simulink model "AeroPlantMIAC_2018a"  (Simulink 9.1)
settings: Solver=VariableStepAuto  StartTime=0.0  StopTime=5  FixedStep=0.01  MaxStep=0.01  RelTol=1e-3  EnableMultiTasking=on
values from neighbouring files (symbols this model uses):
  sigma2e = 0.0    (= 0)    [SA_ACex4_SKRYPT.m]
  Ta = 0.005    [SA_ACex4_SKRYPT.m]
  Tc = 0.001    [SA_ACex4_SKRYPT.m]
  Yr = 0.15    [SA_ACex4_SKRYPT.m]
undefined symbols (not defined in the file or in its folder): T, wr
libraries: simulink x1
settings Model: Creator=Gebruiker  LastModifiedBy=Adam
settings DataIOCC: LimitDataPoints=on  SignalLoggingSaveFormat=ModelDataLogs
settings OptimizationCC: InitFltsAndDblsToZero=on
settings DebuggingCC: SaveWithParameterizedLinksMsg=none  SignalResolutionControl=TryResolveAllWithWarning  SolverPrmCheckMsg=warning  MultiTaskDSMMsg=warning  MultiTaskCondExecSysMsg=none  FcnCallInpInsideContextMsg=warning
settings SFSimCC: SimUseLocalCustomCode=on
settings RTWCC: RTWUseLocalCustomCode=on
settings GRTTargetCC: TargetFcnLib=ansi_tfl_tmw.mat
settings ConfigComp: CovExternalEMLEnable=on

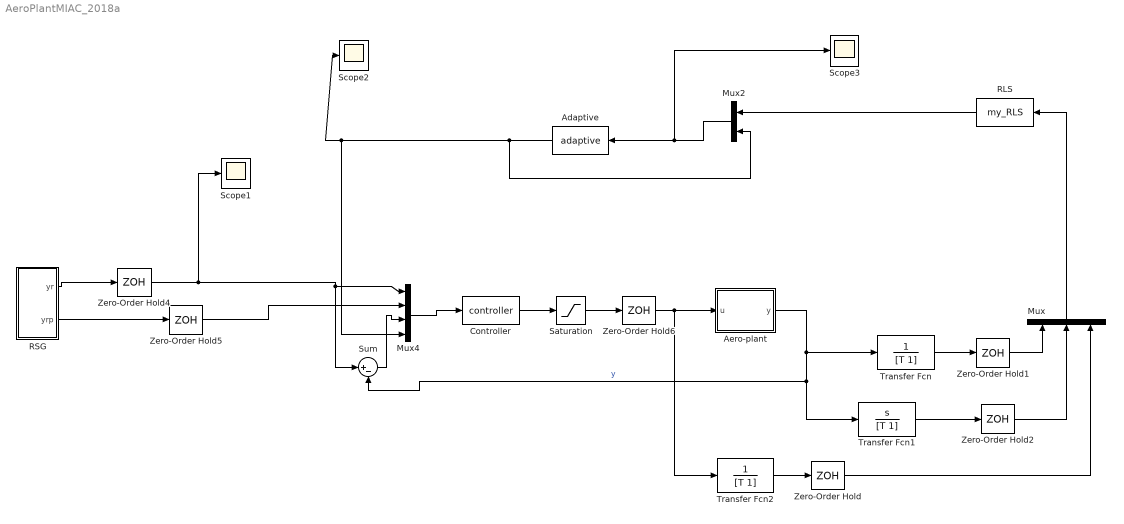
== system AeroPlantMIAC_2018a ==
  Adaptive : MATLABFcn  MATLABFcn=adaptive
  Aero-plant : Subsystem
  Controller : MATLABFcn  MATLABFcn=controller  OutputDimensions=1
  Mux : Mux  Inputs=3
  Mux2 : Mux  Inputs=[2 3]
  Mux4 : Mux
  RLS : MATLABFcn  MATLABFcn=my_RLS  OutputDimensions=2
  RSG : Subsystem
  Saturation : Saturate  UpperLimit=pi/2  LowerLimit=-pi/2
  Scope1 : Scope
  Scope2 : Scope
  Scope3 : Scope
  Sum : Sum  Inputs=|+-
  Transfer Fcn : TransferFcn  Numerator=[0 1]  Denominator=[T 1]
  Transfer Fcn1 : TransferFcn  Numerator=[1 0]  Denominator=[T 1]
  Transfer Fcn2 : TransferFcn  Numerator=[0 1]  Denominator=[T 1]
  Zero-Order Hold : ZeroOrderHold  SampleTime=Ta
  Zero-Order Hold1 : ZeroOrderHold  SampleTime=Ta
  Zero-Order Hold2 : ZeroOrderHold  SampleTime=Ta
  Zero-Order Hold4 : ZeroOrderHold  SampleTime=Tc
  Zero-Order Hold5 : ZeroOrderHold  SampleTime=Tc
  Zero-Order Hold6 : ZeroOrderHold  SampleTime=Tc
  wires:
  Aero-plant/1(y) -> Transfer Fcn1/1, Sum/2, Transfer Fcn/1  "y"
  Mux/1 -> RLS/1
  RSG/2(yrp) -> Zero-Order Hold5/1
  Zero-Order Hold/1 -> Mux/3
  Zero-Order Hold1/1 -> Mux/1
  Zero-Order Hold2/1 -> Mux/2
  RSG/1(yr) -> Zero-Order Hold4/1
  Controller/1 -> Saturation/1
  Adaptive/1 -> Mux4/4, Scope2/1, Mux2/2
  Mux2/1 -> Adaptive/1, Scope3/1
  Sum/1 -> Mux4/3
  RLS/1 -> Mux2/1
  Zero-Order Hold4/1 -> Mux4/1, Sum/1, Scope1/1
  Zero-Order Hold5/1 -> Mux4/2
  Saturation/1 -> Zero-Order Hold6/1
  Zero-Order Hold6/1 -> Aero-plant/1(u), Transfer Fcn2/1
  Transfer Fcn1/1 -> Zero-Order Hold2/1
  Transfer Fcn/1 -> Zero-Order Hold1/1
  Transfer Fcn2/1 -> Zero-Order Hold/1
  Mux4/1 -> Controller/1

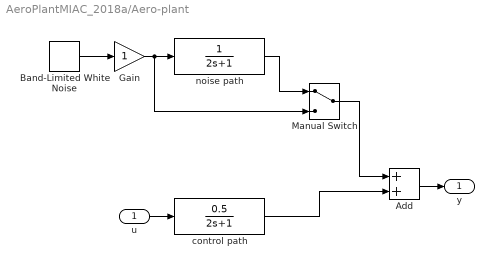
== system AeroPlantMIAC_2018a/Aero-plant ==
  u : Inport
  Add : Sum
  Band-Limited White Noise : simulink/Sources/Band-Limited White Noise  Cov=[sigma2e*Tc]  Ts=Tc  seed=[23341]
  Gain : Gain
  Manual Switch : ManualSwitch
  control path : TransferFcn  Numerator=[0.5]  Denominator=[2 1]
  noise path : TransferFcn  Denominator=[2 1]
  y : Outport
  wires:
  control path/1 -> Add/2
  Band-Limited White Noise/1 -> Gain/1
  Gain/1 -> Manual Switch/2, noise path/1
  Add/1 -> y/1
  u/1 -> control path/1
  noise path/1 -> Manual Switch/1
  Manual Switch/1 -> Add/1

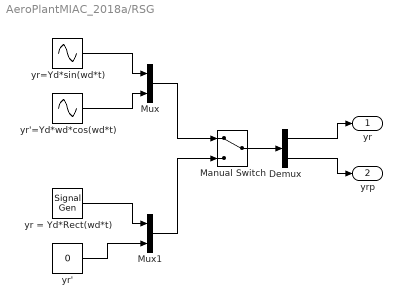
== system AeroPlantMIAC_2018a/RSG ==
  Demux : Demux  Outputs=2
  Manual Switch : ManualSwitch
  Mux : Mux  Inputs=2
  Mux1 : Mux  Inputs=2
  yr = Yd*Rect(wd*t) : SignalGenerator  WaveForm=square  Amplitude=Yr  Frequency=wr  Units=rad/sec
  yr' : Constant  Value=0
  yr'=Yd*wd*cos(wd*t) : Sin  Amplitude=Yr*wr  Frequency=wr  Phase=pi/2  SampleTime=0
  yr=Yd*sin(wd*t) : Sin  Amplitude=Yr  Frequency=wr  SampleTime=0
  yr : Outport
  yrp : Outport  Port=2
  wires:
  yr=Yd*sin(wd*t)/1 -> Mux/1
  yr'=Yd*wd*cos(wd*t)/1 -> Mux/2
  yr = Yd*Rect(wd*t)/1 -> Mux1/1
  yr'/1 -> Mux1/2
  Mux/1 -> Manual Switch/1
  Mux1/1 -> Manual Switch/2
  Manual Switch/1 -> Demux/1
  Demux/1 -> yr/1
  Demux/2 -> yrp/1
